simulink model "lab6_2"  (R2021a)
settings: Solver=VariableStepAuto  StartTime=0.0  StopTime=10.0  RelTol=1e-3
settings Model: Creator=Luka  LastModifiedBy=Luka

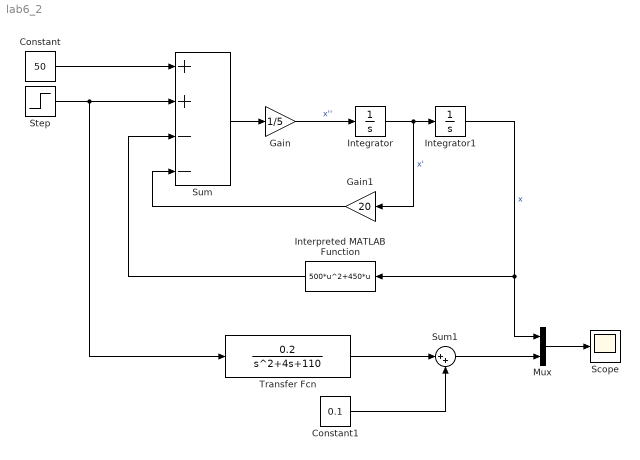
== system lab6_2 ==
  Constant : Constant  Value=50
  Constant1 : Constant  Value=0.1
  Gain : Gain  Gain=1/5
  Gain1 : Gain  Gain=20
  Integrator : Integrator
  Integrator1 : Integrator
  Interpreted MATLAB Function : MATLABFcn  MATLABFcn=500*u^2+450*u
  Mux : Mux  Inputs=2
  Scope : Scope
  Step : Step  Time=5  After=25  SampleTime=0
  Sum : Sum  Inputs=++--
  Sum1 : Sum  Inputs=|++
  Transfer Fcn : TransferFcn  Numerator=[0.2]  Denominator=[1 4 110]
  wires:
  Integrator/1 -> Gain1/1, Integrator1/1  "x'"
  Integrator1/1 -> Mux/1, Interpreted MATLAB Function/1  "x"
  Gain/1 -> Integrator/1  "x''"
  Sum/1 -> Gain/1
  Constant/1 -> Sum/1
  Step/1 -> Transfer Fcn/1, Sum/2
  Gain1/1 -> Sum/4
  Interpreted MATLAB Function/1 -> Sum/3
  Transfer Fcn/1 -> Sum1/1
  Constant1/1 -> Sum1/2
  Sum1/1 -> Mux/2
  Mux/1 -> Scope/1
